simulink model "F16ASYM_Controlled_AoA"  (R2012b)
settings: Solver=ode3  SolverMode=SingleTasking  StartTime=0.0  StopTime=inf  FixedStep=T_sim  RelTol=1e-3
InitFcn:
  | load('NN_c_weights_Last_stable.mat')
values from neighbouring files (symbols this model uses):
  K_b_AoA = params(3)    [Cost_function.m]
  K_b_q = params(4)    [Cost_function.m]
  learning = 20    [Scheduling_desing.m]
  Model_used_flag = 1    [Scheduling_desing.m]
  reg_param = 0.5    [Scheduling_desing.m]
  T_sim = 0.02    [Scheduling_desing.m]
  tau_AoA = params(1)    [Cost_function.m]
  tau_q = params(2)    [Cost_function.m]
  Theta_1_roll_last = [0.00183613313267 0.00115998993235 0.0006676025148 0.00194921904952 0.00134963559861 0.00034352059664 0.000447169388141 0.00146749660935 0.00110199952389 7.77922383894e-05 0.00109492833348 0.00192687590535 ... (360 elements, 30x12)]    [NN_i_weights_LAST_STABLE.mat]
  Theta_2_roll_last = [0.000469743069697 0.000355923851088 0.00180035760697 0.00191855117771 0.00118851504447 0.0013331642065 0.0013164316578 0.000643981263341 0.00176817665434 0.000113802099363 0.000426534542462 0.00113815782354 ... (620 elements, 20x31)]    [NN_i_weights_LAST_STABLE.mat]
  Theta_3_roll_last = [9.62071520568e-05 -0.000389870886846 2.08260845013e-05 0.000140787743673 -0.000917525755397 -0.0014324207578 -0.00154701573815 -0.00131544476264 -0.00101205584381 5.06515794689e-05 -0.00111443483676 -0.00143957416141 ... (21 elements, 1x21)]    [NN_i_weights_LAST_STABLE.mat]
  V_long_lastA_w_z = [0.352826086601 -0.253633004548 -0.642535042878 0.237749930435 -0.618390629538 0.858074761295 0.268211230628 -0.448715080196 -0.0406384631192 0.401147605577 0.60598427709 0.0500551915851 ... (300 elements, 30x10)]    [NN_i_weights_LAST_STABLE.mat]
  V_long_lastAoA = [0.0774300162379 0.0911421319631 0.0352371192557 0.0542170286952 0.0651171200844 0.0177112012707 0.0982957728448 0.000259994642558 0.0194724569123 0.0466321328252 0.0556687953852 0.0252668067142 ... (300 elements, 30x10)]    [NN_i_weights_LAST_STABLE.mat]
  V_roll_last = [0.0540918675943 0.0557493347212 0.0839792276608 0.0460576391794 0.0671229058124 0.100220403067 0.0722493281881 0.0648875457457 0.00447599349201 0.0607299103823 0.0488037966361 0.0176785979393 ... (360 elements, 30x12)]    [NN_i_weights_LAST_STABLE.mat]
  V_yaw_last = [0.0965149149679 0.00833616709545 0.0365734360076 0.0523944217566 0.00790252078455 0.0700053845887 0.0345164868709 0.0111568465295 0.094060639546 0.0205483560006 0.000798047494256 0.0862769385758 ... (360 elements, 30x12)]    [NN_i_weights_LAST_STABLE.mat]
  velocity = M_eval_sche(I,J)*a    [Scheduling_desing.m]
  W_long_lastA_w_z = [-0.0522913429974 0.00385484301394 -0.00465489482472 -0.0139416219936 0.00295196421483 -0.013027768541 0.00585545058915 0.00278802233571 -0.00906272782329 -0.000396112031465 0.00405849743321 0.00509668457818 ... (31 elements, 1x31)]    [NN_i_weights_LAST_STABLE.mat]
  W_long_lastAoA = [-0.0192589013922 0.00873109909713 0.00432649597332 0.0420946902441 0.0293366820194 0.0351497798191 0.0234952374236 0.0360841187718 0.0112233388211 0.030147202199 0.0369533138617 0.00218839076415 ... (31 elements, 1x31)]    [NN_i_weights_LAST_STABLE.mat]
  W_roll_last = [-0.0006515532842 0.000535485585715 0.000550946920743 0.000806030945453 0.00045976209382 0.00065557954304 0.000945902185602 0.00070191398535 0.000635215543728 4.66501377412e-05 0.000597079583757 0.000485790566765 ... (31 elements, 1x31)]    [NN_i_weights_LAST_STABLE.mat]
  W_yaw_last = [-4.34263633305e-05 8.83823048922e-05 1.65575463724e-05 3.60293102233e-05 5.19752447623e-05 7.06399280852e-06 7.02425975821e-05 3.62680255076e-05 1.29996379937e-05 8.05072914397e-05 2.39941870661e-05 2.52427840574e-06 ... (31 elements, 1x31)]    [NN_i_weights_LAST_STABLE.mat]
undefined symbols (not defined in the file or in its folder): a1, alpha_map_eval, B, beta_map_eval, C_L_0, DiscIntNeverNeededParam, fi_flag_Simulink, G_eval, H_sq, H_sq_autotrim, k_B, m_B, M_sq, M_sq_autotrim, sigbuilder_block, Stall_curve, trim_control, trim_state, trim_throttle, V_Comp_A_w_z_last, V_Comp_last, V_roll_lastMOD, W_Comp_A_w_z_last, W_Comp_last, W_roll_lastMOD
libraries: Adaptive_FaultTolerantControl x43, dspsigops x29, F16_Actuator_Library x14, simulink x8, aerolibatmos2 x7, dsparch4 x6, simulink_extras x5, aerolibtransform2 x5, qcatlib x4, dspmtrx3 x3, dspvision x2, dspsnks4 x2
(part 7 of 11)

== system F16ASYM_Controlled_AoA/Control allocator/Control allocator: RECONFIG/Blockades logic: Limits injetor/Block AT SUPERIOR LIMIT ==
  Limit : Inport
  Blockades : Inport  Port=2
  Demux : Demux  Outputs=7
  Mux2 : Mux  Inputs=7
  Selector : Selector  InputPortWidth=7  IndexOptions=Index vector (dialog)  Indices=1  OutputSizes=1
  Selector1 : Selector  InputPortWidth=7  IndexOptions=Index vector (dialog)  Indices=2  OutputSizes=1
  Selector2 : Selector  InputPortWidth=7  IndexOptions=Index vector (dialog)  Indices=3  OutputSizes=1
  Selector3 : Selector  InputPortWidth=7  IndexOptions=Index vector (dialog)  Indices=4  OutputSizes=1
  Selector4 : Selector  InputPortWidth=7  IndexOptions=Index vector (dialog)  Indices=5  OutputSizes=1
  Selector5 : Selector  InputPortWidth=7  IndexOptions=Index vector (dialog)  Indices=6  OutputSizes=1
  Selector6 : Selector  InputPortWidth=7  IndexOptions=Index vector (dialog)  Indices=7  OutputSizes=1
  Switch{,1..6} (7 alike) : Switch  Threshold=0.5
  isNaN{,1..6} (7 alike) : RelationalOperator  Operator=isNaN  OutDataTypeStr=boolean
  Reconfig limits : Outport
  wires:
  Switch6/1 -> Mux2/7
  Switch5/1 -> Mux2/6  "LEF_L"
  Switch4/1 -> Mux2/5  "Rudder"
  Switch3/1 -> Mux2/4  "Aileron_R"
  Switch2/1 -> Mux2/3  "Aileron_L"
  Switch1/1 -> Mux2/2
  Switch/1 -> Mux2/1  "Elevator_L"
  Blockades/1 -> [Blockades]
  Mux2/1 -> Reconfig limits/1
  Limit/1 -> Demux/1
  Selector6/1 -> isNaN6/1, Switch6/3
  Demux/7 -> Switch6/1
  isNaN6/1 -> Switch6/2
  [Blockades] -> Selector6/1
  Selector5/1 -> isNaN5/1, Switch5/3
  Demux/6 -> Switch5/1
  isNaN5/1 -> Switch5/2
  [Blockades] -> Selector5/1
  Selector4/1 -> isNaN4/1, Switch4/3
  Demux/5 -> Switch4/1
  isNaN4/1 -> Switch4/2
  [Blockades] -> Selector4/1
  Selector3/1 -> isNaN3/1, Switch3/3
  Demux/4 -> Switch3/1
  isNaN3/1 -> Switch3/2
  [Blockades] -> Selector3/1
  Selector2/1 -> isNaN2/1, Switch2/3
  Demux/3 -> Switch2/1
  isNaN2/1 -> Switch2/2
  [Blockades] -> Selector2/1
  Selector1/1 -> isNaN1/1, Switch1/3
  Demux/2 -> Switch1/1
  isNaN1/1 -> Switch1/2
  [Blockades] -> Selector1/1
  Selector/1 -> isNaN/1, Switch/3
  Demux/1 -> Switch/1
  isNaN/1 -> Switch/2
  [Blockades] -> Selector/1

== system F16ASYM_Controlled_AoA/Control allocator/Control allocator: RECONFIG/Blockades logic: Limits injetor/Block NOW INFERIOR LIMIT ==
  Limit : Inport
  Blockade now : Inport  Port=2
  Last deflection (abs) : Inport  Port=3
  Demux : Demux  Outputs=7
  Mux2 : Mux  Inputs=7
  Selector1 : Selector  InputPortWidth=7  IndexOptions=Index vector (dialog)  Indices=1  OutputSizes=1
  Selector10 : Selector  InputPortWidth=7  IndexOptions=Index vector (dialog)  Indices=4  OutputSizes=1
  Selector11 : Selector  InputPortWidth=7  IndexOptions=Index vector (dialog)  Indices=5  OutputSizes=1
  Selector12 : Selector  InputPortWidth=7  IndexOptions=Index vector (dialog)  Indices=6  OutputSizes=1
  Selector13 : Selector  InputPortWidth=7  IndexOptions=Index vector (dialog)  Indices=7  OutputSizes=1
  Selector14 : Selector  InputPortWidth=7  IndexOptions=Index vector (dialog)  Indices=7  OutputSizes=1
  Selector2 : Selector  InputPortWidth=7  IndexOptions=Index vector (dialog)  Indices=2  OutputSizes=1
  Selector3 : Selector  InputPortWidth=7  IndexOptions=Index vector (dialog)  Indices=3  OutputSizes=1
  Selector4 : Selector  InputPortWidth=7  IndexOptions=Index vector (dialog)  Indices=4  OutputSizes=1
  Selector5 : Selector  InputPortWidth=7  IndexOptions=Index vector (dialog)  Indices=5  OutputSizes=1
  Selector6 : Selector  InputPortWidth=7  IndexOptions=Index vector (dialog)  Indices=6  OutputSizes=1
  Selector7 : Selector  InputPortWidth=7  IndexOptions=Index vector (dialog)  Indices=1  OutputSizes=1
  Selector8 : Selector  InputPortWidth=7  IndexOptions=Index vector (dialog)  Indices=2  OutputSizes=1
  Selector9 : Selector  InputPortWidth=7  IndexOptions=Index vector (dialog)  Indices=3  OutputSizes=1
  Switch{7..13} (7 alike) : Switch  Threshold=0.5
  Reconfig limits : Outport
  wires:
  Mux2/1 -> Reconfig limits/1
  Limit/1 -> Demux/1
  Selector13/1 -> Switch13/2
  [Blockade_now] -> Selector13/1
  Demux/7 -> Switch13/3
  Selector12/1 -> Switch12/2
  [Blockade_now] -> Selector12/1
  Demux/6 -> Switch12/3  "LEF_L"
  Selector11/1 -> Switch11/2
  [Blockade_now] -> Selector11/1
  Demux/5 -> Switch11/3  "Rudder"
  Selector10/1 -> Switch10/2
  [Blockade_now] -> Selector10/1
  Demux/4 -> Switch10/3  "Aileron_R"
  Selector9/1 -> Switch9/2
  [Blockade_now] -> Selector9/1
  Selector8/1 -> Switch8/2
  [Blockade_now] -> Selector8/1
  Demux/2 -> Switch8/3
  Selector7/1 -> Switch7/2
  [Blockade_now] -> Selector7/1
  Demux/1 -> Switch7/3  "Elevator_L"
  Blockade now/1 -> [Blockade_now]
  Last deflection (abs)/1 -> [Actual_defle]
  Demux/3 -> Switch9/3
  Switch7/1 -> Mux2/1
  Switch8/1 -> Mux2/2
  Switch9/1 -> Mux2/3
  Switch10/1 -> Mux2/4
  Switch11/1 -> Mux2/5
  Switch12/1 -> Mux2/6
  Switch13/1 -> Mux2/7
  [Actual_defle] -> Selector1/1
  Selector1/1 -> Switch7/1
  [Actual_defle] -> Selector2/1
  Selector2/1 -> Switch8/1
  Selector3/1 -> Switch9/1
  [Actual_defle] -> Selector3/1
  Selector4/1 -> Switch10/1
  [Actual_defle] -> Selector4/1
  Selector5/1 -> Switch11/1
  [Actual_defle] -> Selector5/1
  Selector6/1 -> Switch12/1
  [Actual_defle] -> Selector6/1
  Selector14/1 -> Switch13/1
  [Actual_defle] -> Selector14/1

== system F16ASYM_Controlled_AoA/Control allocator/Control allocator: RECONFIG/Blockades logic: Limits injetor/Block NOW SUPERIOR LIMIT ==
  Limit : Inport
  Blockade now : Inport  Port=2
  Last deflection (abs) : Inport  Port=3
  Demux : Demux  Outputs=7
  Mux2 : Mux  Inputs=7
  Selector1 : Selector  InputPortWidth=7  IndexOptions=Index vector (dialog)  Indices=1  OutputSizes=1
  Selector10 : Selector  InputPortWidth=7  IndexOptions=Index vector (dialog)  Indices=4  OutputSizes=1
  Selector11 : Selector  InputPortWidth=7  IndexOptions=Index vector (dialog)  Indices=5  OutputSizes=1
  Selector12 : Selector  InputPortWidth=7  IndexOptions=Index vector (dialog)  Indices=6  OutputSizes=1
  Selector13 : Selector  InputPortWidth=7  IndexOptions=Index vector (dialog)  Indices=7  OutputSizes=1
  Selector14 : Selector  InputPortWidth=7  IndexOptions=Index vector (dialog)  Indices=7  OutputSizes=1
  Selector2 : Selector  InputPortWidth=7  IndexOptions=Index vector (dialog)  Indices=2  OutputSizes=1
  Selector3 : Selector  InputPortWidth=7  IndexOptions=Index vector (dialog)  Indices=3  OutputSizes=1
  Selector4 : Selector  InputPortWidth=7  IndexOptions=Index vector (dialog)  Indices=4  OutputSizes=1
  Selector5 : Selector  InputPortWidth=7  IndexOptions=Index vector (dialog)  Indices=5  OutputSizes=1
  Selector6 : Selector  InputPortWidth=7  IndexOptions=Index vector (dialog)  Indices=6  OutputSizes=1
  Selector7 : Selector  InputPortWidth=7  IndexOptions=Index vector (dialog)  Indices=1  OutputSizes=1
  Selector8 : Selector  InputPortWidth=7  IndexOptions=Index vector (dialog)  Indices=2  OutputSizes=1
  Selector9 : Selector  InputPortWidth=7  IndexOptions=Index vector (dialog)  Indices=3  OutputSizes=1
  Switch{7..13} (7 alike) : Switch  Threshold=0.5
  Reconfig limits : Outport
  wires:
  [Actual_defle] -> Selector14/1
  Selector14/1 -> Switch13/1
  [Actual_defle] -> Selector6/1
  Selector6/1 -> Switch12/1
  [Actual_defle] -> Selector5/1
  Selector5/1 -> Switch11/1
  [Actual_defle] -> Selector4/1
  Selector4/1 -> Switch10/1
  [Actual_defle] -> Selector3/1
  Selector3/1 -> Switch9/1
  Selector2/1 -> Switch8/1
  [Actual_defle] -> Selector2/1
  Selector1/1 -> Switch7/1
  [Actual_defle] -> Selector1/1
  Switch13/1 -> Mux2/7
  Switch12/1 -> Mux2/6
  Switch11/1 -> Mux2/5
  Switch10/1 -> Mux2/4
  Switch9/1 -> Mux2/3
  Switch8/1 -> Mux2/2
  Switch7/1 -> Mux2/1
  Demux/3 -> Switch9/3
  Last deflection (abs)/1 -> [Actual_defle]
  Blockade now/1 -> [Blockade_now]
  Demux/1 -> Switch7/3  "Elevator_L"
  [Blockade_now] -> Selector7/1
  Selector7/1 -> Switch7/2
  Demux/2 -> Switch8/3
  [Blockade_now] -> Selector8/1
  Selector8/1 -> Switch8/2
  [Blockade_now] -> Selector9/1
  Selector9/1 -> Switch9/2
  Demux/4 -> Switch10/3  "Aileron_R"
  [Blockade_now] -> Selector10/1
  Selector10/1 -> Switch10/2
  Demux/5 -> Switch11/3  "Rudder"
  [Blockade_now] -> Selector11/1
  Selector11/1 -> Switch11/2
  Demux/6 -> Switch12/3  "LEF_L"
  [Blockade_now] -> Selector12/1
  Selector12/1 -> Switch12/2
  Demux/7 -> Switch13/3
  [Blockade_now] -> Selector13/1
  Selector13/1 -> Switch13/2
  Limit/1 -> Demux/1
  Mux2/1 -> Reconfig limits/1

== system F16ASYM_Controlled_AoA/Control allocator/Control allocator: RECONFIG/Leading Edge Flap:Symetric deflection/Creating    qbar // ps ==
  alt : Inport
  V : Inport  Port=2
  ISA Atmosphere Model : aerolibatmos2/ISA Atmosphere Model  custom=off  g=9.80665  gamma=1.4  R=287.0531  L=0.0065  h_trop=11000  h_strat=20000  rho0=1.225  P0=101325  T0=288.15
  Math Function1 : Math  Operator=square  SaturateOnIntegerOverflow=on
  Product : Product  Inputs=/*  SaturateOnIntegerOverflow=on  InputSameDT=on  OutDataTypeStr=Inherit: Same as first input
  Product5 : Product  Inputs=**  SaturateOnIntegerOverflow=on  InputSameDT=on  OutDataTypeStr=Inherit: Same as first input
  Terminator : Terminator
  Terminator1 : Terminator
  r2d4 : Gain  Gain=0.5  SaturateOnIntegerOverflow=on  OutDataTypeStr=Inherit: Same as input  ParamDataTypeStr=Inherit: Same as input
  qbar / ps : Outport
  wires:
  alt/1 -> ISA Atmosphere Model/1
  Math Function1/1 -> r2d4/1
  r2d4/1 -> Product5/2
  Product5/1 -> Product/2  "qbar"
  V/1 -> Math Function1/1
  Product/1 -> qbar / ps/1
  ISA Atmosphere Model/4 -> Product5/1
  ISA Atmosphere Model/3 -> Product/1
  ISA Atmosphere Model/1 -> Terminator/1
  ISA Atmosphere Model/2 -> Terminator1/1

== system F16ASYM_Controlled_AoA/Control allocator1/Control allocator: NO RECONF/Leading Edge Flap:Symetric deflection/Creating    qbar // ps ==
  alt : Inport
  V : Inport  Port=2
  ISA Atmosphere Model : aerolibatmos2/ISA Atmosphere Model  custom=off  g=9.80665  gamma=1.4  R=287.0531  L=0.0065  h_trop=11000  h_strat=20000  rho0=1.225  P0=101325  T0=288.15
  Math Function1 : Math  Operator=square  SaturateOnIntegerOverflow=on
  Product : Product  Inputs=/*  SaturateOnIntegerOverflow=on  InputSameDT=on  OutDataTypeStr=Inherit: Same as first input
  Product5 : Product  Inputs=**  SaturateOnIntegerOverflow=on  InputSameDT=on  OutDataTypeStr=Inherit: Same as first input
  Terminator : Terminator
  Terminator1 : Terminator
  r2d4 : Gain  Gain=0.5  SaturateOnIntegerOverflow=on  OutDataTypeStr=Inherit: Same as input  ParamDataTypeStr=Inherit: Same as input
  qbar / ps : Outport
  wires:
  ISA Atmosphere Model/2 -> Terminator1/1
  ISA Atmosphere Model/1 -> Terminator/1
  ISA Atmosphere Model/3 -> Product/1
  ISA Atmosphere Model/4 -> Product5/1
  Product/1 -> qbar / ps/1
  V/1 -> Math Function1/1
  Product5/1 -> Product/2  "qbar"
  r2d4/1 -> Product5/2
  Math Function1/1 -> r2d4/1
  alt/1 -> ISA Atmosphere Model/1

== system F16ASYM_Controlled_AoA/Control allocator1/Control allocator: RECONFIG/Blockades logic: Limits injetor/1st order model ==
  y_in : Inport
  Add : Sum  Inputs=|+-
  Integrator : Integrator  InitialCondition=y_i
  K_ref : Gain  Gain=K_ref
  y_out : Outport
  wires:
  Integrator/1 -> Add/2, y_out/1
  K_ref/1 -> Integrator/1
  Add/1 -> K_ref/1
  y_in/1 -> Add/1

== system F16ASYM_Controlled_AoA/Control allocator1/Control allocator: RECONFIG/Blockades logic: Limits injetor/1st order model1 ==
  y_in : Inport
  Add : Sum  Inputs=|+-
  Integrator : Integrator  InitialCondition=y_i
  K_ref : Gain  Gain=K_ref
  y_out : Outport
  wires:
  y_in/1 -> Add/1
  Add/1 -> K_ref/1
  K_ref/1 -> Integrator/1
  Integrator/1 -> y_out/1, Add/2

== system F16ASYM_Controlled_AoA/Control allocator1/Control allocator: RECONFIG/Blockades logic: Limits injetor/Block AT INFERIOR LIMIT ==
  Limit : Inport
  Blockades : Inport  Port=2
  Demux : Demux  Outputs=7
  Logical Operator : Logic  Operator=NOT  IconShape=distinctive  AllPortsSameDT=off  OutDataTypeStr=boolean
  Mux1 : Mux  Inputs=7
  Mux2 : Mux  Inputs=7
  Selector : Selector  InputPortWidth=7  IndexOptions=Index vector (dialog)  Indices=1  OutputSizes=1
  Selector1 : Selector  InputPortWidth=7  IndexOptions=Index vector (dialog)  Indices=2  OutputSizes=1
  Selector2 : Selector  InputPortWidth=7  IndexOptions=Index vector (dialog)  Indices=3  OutputSizes=1
  Selector3 : Selector  InputPortWidth=7  IndexOptions=Index vector (dialog)  Indices=4  OutputSizes=1
  Selector4 : Selector  InputPortWidth=7  IndexOptions=Index vector (dialog)  Indices=5  OutputSizes=1
  Selector5 : Selector  InputPortWidth=7  IndexOptions=Index vector (dialog)  Indices=6  OutputSizes=1
  Selector6 : Selector  InputPortWidth=7  IndexOptions=Index vector (dialog)  Indices=7  OutputSizes=1
  Switch{,1..6} (7 alike) : Switch  Threshold=0.5
  isNaN{,1..6} (7 alike) : RelationalOperator  Operator=isNaN  OutDataTypeStr=boolean
  Reconfig limits : Outport
  Surf blocked : Outport  Port=2
  wires:
  [Blockades] -> Selector/1
  isNaN/1 -> [left_elev], Switch/2
  Demux/1 -> Switch/1
  Selector/1 -> Switch/3, isNaN/1
  [Blockades] -> Selector1/1
  isNaN1/1 -> [right_elev], Switch1/2
  Demux/2 -> Switch1/1
  Selector1/1 -> Switch1/3, isNaN1/1
  [Blockades] -> Selector2/1
  isNaN2/1 -> Switch2/2, [left_ail]
  Demux/3 -> Switch2/1
  Selector2/1 -> Switch2/3, isNaN2/1
  [Blockades] -> Selector3/1
  isNaN3/1 -> [right_ail], Switch3/2
  Demux/4 -> Switch3/1
  Selector3/1 -> Switch3/3, isNaN3/1
  [Blockades] -> Selector4/1
  isNaN4/1 -> [rudder], Switch4/2
  Demux/5 -> Switch4/1
  Selector4/1 -> Switch4/3, isNaN4/1
  [Blockades] -> Selector5/1
  isNaN5/1 -> [left_LEF], Switch5/2
  Demux/6 -> Switch5/1
  Selector5/1 -> Switch5/3, isNaN5/1
  [Blockades] -> Selector6/1
  isNaN6/1 -> [rith_LEF], Switch6/2
  Demux/7 -> Switch6/1
  Selector6/1 -> Switch6/3, isNaN6/1
  Limit/1 -> Demux/1
  Mux2/1 -> Reconfig limits/1
  Blockades/1 -> [Blockades]
  Switch/1 -> Mux2/1  "Elevator_L"
  Switch1/1 -> Mux2/2
  Switch2/1 -> Mux2/3  "Aileron_L"
  Switch3/1 -> Mux2/4  "Aileron_R"
  Switch4/1 -> Mux2/5  "Rudder"
  Switch5/1 -> Mux2/6  "LEF_L"
  Switch6/1 -> Mux2/7
  [left_elev] -> Mux1/1
  Mux1/1 -> Logical Operator/1
  [right_elev] -> Mux1/2
  [left_ail] -> Mux1/3
  [right_ail] -> Mux1/4
  [rudder] -> Mux1/5
  [left_LEF] -> Mux1/6
  [rith_LEF] -> Mux1/7
  Logical Operator/1 -> Surf blocked/1

== system F16ASYM_Controlled_AoA/Control allocator1/Control allocator: RECONFIG/Blockades logic: Limits injetor/Block AT SUPERIOR LIMIT ==
  Limit : Inport
  Blockades : Inport  Port=2
  Demux : Demux  Outputs=7
  Mux2 : Mux  Inputs=7
  Selector : Selector  InputPortWidth=7  IndexOptions=Index vector (dialog)  Indices=1  OutputSizes=1
  Selector1 : Selector  InputPortWidth=7  IndexOptions=Index vector (dialog)  Indices=2  OutputSizes=1
  Selector2 : Selector  InputPortWidth=7  IndexOptions=Index vector (dialog)  Indices=3  OutputSizes=1
  Selector3 : Selector  InputPortWidth=7  IndexOptions=Index vector (dialog)  Indices=4  OutputSizes=1
  Selector4 : Selector  InputPortWidth=7  IndexOptions=Index vector (dialog)  Indices=5  OutputSizes=1
  Selector5 : Selector  InputPortWidth=7  IndexOptions=Index vector (dialog)  Indices=6  OutputSizes=1
  Selector6 : Selector  InputPortWidth=7  IndexOptions=Index vector (dialog)  Indices=7  OutputSizes=1
  Switch{,1..6} (7 alike) : Switch  Threshold=0.5
  isNaN{,1..6} (7 alike) : RelationalOperator  Operator=isNaN  OutDataTypeStr=boolean
  Reconfig limits : Outport
  wires:
  Switch6/1 -> Mux2/7
  Switch5/1 -> Mux2/6  "LEF_L"
  Switch4/1 -> Mux2/5  "Rudder"
  Switch3/1 -> Mux2/4  "Aileron_R"
  Switch2/1 -> Mux2/3  "Aileron_L"
  Switch1/1 -> Mux2/2
  Switch/1 -> Mux2/1  "Elevator_L"
  Blockades/1 -> [Blockades]
  Mux2/1 -> Reconfig limits/1
  Limit/1 -> Demux/1
  Selector6/1 -> isNaN6/1, Switch6/3
  Demux/7 -> Switch6/1
  isNaN6/1 -> Switch6/2
  [Blockades] -> Selector6/1
  Selector5/1 -> isNaN5/1, Switch5/3
  Demux/6 -> Switch5/1
  isNaN5/1 -> Switch5/2
  [Blockades] -> Selector5/1
  Selector4/1 -> isNaN4/1, Switch4/3
  Demux/5 -> Switch4/1
  isNaN4/1 -> Switch4/2
  [Blockades] -> Selector4/1
  Selector3/1 -> isNaN3/1, Switch3/3
  Demux/4 -> Switch3/1
  isNaN3/1 -> Switch3/2
  [Blockades] -> Selector3/1
  Selector2/1 -> isNaN2/1, Switch2/3
  Demux/3 -> Switch2/1
  isNaN2/1 -> Switch2/2
  [Blockades] -> Selector2/1
  Selector1/1 -> isNaN1/1, Switch1/3
  Demux/2 -> Switch1/1
  isNaN1/1 -> Switch1/2
  [Blockades] -> Selector1/1
  Selector/1 -> isNaN/1, Switch/3
  Demux/1 -> Switch/1
  isNaN/1 -> Switch/2
  [Blockades] -> Selector/1

== system F16ASYM_Controlled_AoA/Control allocator1/Control allocator: RECONFIG/Blockades logic: Limits injetor/Block NOW INFERIOR LIMIT ==
  Limit : Inport
  Blockade now : Inport  Port=2
  Last deflection (abs) : Inport  Port=3
  Demux : Demux  Outputs=7
  Mux2 : Mux  Inputs=7
  Sample and Hold{,1..7} (8 alike) : dspsigops/Sample and Hold  trig=Rising edge  initCond=trim_control(1)  latchinput=off
  Selector1 : Selector  InputPortWidth=7  IndexOptions=Index vector (dialog)  Indices=1  OutputSizes=1
  Selector10 : Selector  InputPortWidth=7  IndexOptions=Index vector (dialog)  Indices=4  OutputSizes=1
  Selector11 : Selector  InputPortWidth=7  IndexOptions=Index vector (dialog)  Indices=5  OutputSizes=1
  Selector12 : Selector  InputPortWidth=7  IndexOptions=Index vector (dialog)  Indices=6  OutputSizes=1
  Selector13 : Selector  InputPortWidth=7  IndexOptions=Index vector (dialog)  Indices=7  OutputSizes=1
  Selector14 : Selector  InputPortWidth=7  IndexOptions=Index vector (dialog)  Indices=7  OutputSizes=1
  Selector15 : Selector  InputPortWidth=7  IndexOptions=Index vector (dialog)  Indices=1  OutputSizes=1
  Selector2 : Selector  InputPortWidth=7  IndexOptions=Index vector (dialog)  Indices=2  OutputSizes=1
  Selector3 : Selector  InputPortWidth=7  IndexOptions=Index vector (dialog)  Indices=3  OutputSizes=1
  Selector4 : Selector  InputPortWidth=7  IndexOptions=Index vector (dialog)  Indices=4  OutputSizes=1
  Selector5 : Selector  InputPortWidth=7  IndexOptions=Index vector (dialog)  Indices=5  OutputSizes=1
  Selector6 : Selector  InputPortWidth=7  IndexOptions=Index vector (dialog)  Indices=6  OutputSizes=1
  Selector7 : Selector  InputPortWidth=7  IndexOptions=Index vector (dialog)  Indices=1  OutputSizes=1
  Selector8 : Selector  InputPortWidth=7  IndexOptions=Index vector (dialog)  Indices=2  OutputSizes=1
  Selector9 : Selector  InputPortWidth=7  IndexOptions=Index vector (dialog)  Indices=3  OutputSizes=1
  Switch{1,7..13} (8 alike) : Switch  Threshold=0.5
  Reconfig limits : Outport
  wires:
  Mux2/1 -> Reconfig limits/1
  Limit/1 -> Demux/1
  Selector13/1 -> Sample and Hold7/Trigger, Switch13/2
  [Blockade_now] -> Selector13/1
  Demux/7 -> Switch13/3
  Selector12/1 -> Switch12/2, Sample and Hold6/Trigger
  [Blockade_now] -> Selector12/1
  Demux/6 -> Switch12/3  "LEF_L"
  Selector11/1 -> Sample and Hold5/Trigger, Switch11/2
  [Blockade_now] -> Selector11/1
  Demux/5 -> Switch11/3  "Rudder"
  Selector10/1 -> Switch10/2, Sample and Hold4/Trigger
  [Blockade_now] -> Selector10/1
  Demux/4 -> Switch10/3  "Aileron_R"
  Selector9/1 -> Sample and Hold2/Trigger, Switch9/2
  [Blockade_now] -> Selector9/1
  Selector8/1 -> Sample and Hold3/Trigger, Switch8/2
  [Blockade_now] -> Selector8/1
  Demux/2 -> Switch8/3
  Selector7/1 -> Sample and Hold1/Trigger, Switch7/2
  [Blockade_now] -> Selector7/1
  Demux/1 -> Switch7/3  "Elevator_L"
  Blockade now/1 -> [Blockade_now]
  Last deflection (abs)/1 -> [Actual_defle]
  Demux/3 -> Switch9/3
  Switch7/1 -> Mux2/1
  Switch8/1 -> Mux2/2
  Switch9/1 -> Mux2/3
  Switch10/1 -> Mux2/4
  Switch11/1 -> Mux2/5
  Switch12/1 -> Mux2/6
  Switch13/1 -> Mux2/7
  [Actual_defle] -> Selector1/1
  Selector1/1 -> Sample and Hold1/1
  [Actual_defle] -> Selector2/1
  Selector2/1 -> Sample and Hold3/1
  Selector3/1 -> Sample and Hold2/1
  [Actual_defle] -> Selector3/1
  Selector4/1 -> Sample and Hold4/1
  [Actual_defle] -> Selector4/1
  Selector5/1 -> Sample and Hold5/1
  [Actual_defle] -> Selector5/1
  Sample and Hold6/1 -> Switch12/1
  [Actual_defle] -> Selector6/1
  Selector14/1 -> Sample and Hold7/1
  [Actual_defle] -> Selector14/1
  ? -> Switch1/3, Sample and Hold/1  "Elevator_L"
  [Blockade_now] -> Selector15/1
  Sample and Hold/1 -> Switch1/1
  Selector15/1 -> Switch1/2, Sample and Hold/Trigger
  Sample and Hold1/1 -> Switch7/1
  Sample and Hold2/1 -> Switch9/1
  Sample and Hold3/1 -> Switch8/1
  Sample and Hold4/1 -> Switch10/1
  Sample and Hold5/1 -> Switch11/1
  Selector6/1 -> Sample and Hold6/1
  Sample and Hold7/1 -> Switch13/1

== system F16ASYM_Controlled_AoA/Control allocator1/Control allocator: RECONFIG/Blockades logic: Limits injetor/Block NOW SUPERIOR LIMIT ==
  Limit : Inport
  Blockade now : Inport  Port=2
  Last deflection (abs) : Inport  Port=3
  Demux : Demux  Outputs=7
  Mux2 : Mux  Inputs=7
  Sample and Hold{,1..7} (8 alike) : dspsigops/Sample and Hold  trig=Rising edge  initCond=trim_control(1)  latchinput=off
  Selector1 : Selector  InputPortWidth=7  IndexOptions=Index vector (dialog)  Indices=1  OutputSizes=1
  Selector10 : Selector  InputPortWidth=7  IndexOptions=Index vector (dialog)  Indices=4  OutputSizes=1
  Selector11 : Selector  InputPortWidth=7  IndexOptions=Index vector (dialog)  Indices=5  OutputSizes=1
  Selector12 : Selector  InputPortWidth=7  IndexOptions=Index vector (dialog)  Indices=6  OutputSizes=1
  Selector13 : Selector  InputPortWidth=7  IndexOptions=Index vector (dialog)  Indices=7  OutputSizes=1
  Selector14 : Selector  InputPortWidth=7  IndexOptions=Index vector (dialog)  Indices=7  OutputSizes=1
  Selector15 : Selector  InputPortWidth=7  IndexOptions=Index vector (dialog)  Indices=1  OutputSizes=1
  Selector2 : Selector  InputPortWidth=7  IndexOptions=Index vector (dialog)  Indices=2  OutputSizes=1
  Selector3 : Selector  InputPortWidth=7  IndexOptions=Index vector (dialog)  Indices=3  OutputSizes=1
  Selector4 : Selector  InputPortWidth=7  IndexOptions=Index vector (dialog)  Indices=4  OutputSizes=1
  Selector5 : Selector  InputPortWidth=7  IndexOptions=Index vector (dialog)  Indices=5  OutputSizes=1
  Selector6 : Selector  InputPortWidth=7  IndexOptions=Index vector (dialog)  Indices=6  OutputSizes=1
  Selector7 : Selector  InputPortWidth=7  IndexOptions=Index vector (dialog)  Indices=1  OutputSizes=1
  Selector8 : Selector  InputPortWidth=7  IndexOptions=Index vector (dialog)  Indices=2  OutputSizes=1
  Selector9 : Selector  InputPortWidth=7  IndexOptions=Index vector (dialog)  Indices=3  OutputSizes=1
  Switch{1,7..13} (8 alike) : Switch  Threshold=0.5
  Reconfig limits : Outport
  wires:
  Sample and Hold7/1 -> Switch13/1
  Selector6/1 -> Sample and Hold6/1
  Sample and Hold5/1 -> Switch11/1
  Sample and Hold4/1 -> Switch10/1
  Sample and Hold3/1 -> Switch8/1
  Sample and Hold2/1 -> Switch9/1
  Sample and Hold1/1 -> Switch7/1
  Selector15/1 -> Sample and Hold/Trigger, Switch1/2
  Sample and Hold/1 -> Switch1/1
  [Blockade_now] -> Selector15/1
  ? -> Sample and Hold/1, Switch1/3  "Elevator_L"
  [Actual_defle] -> Selector14/1
  Selector14/1 -> Sample and Hold7/1
  [Actual_defle] -> Selector6/1
  Sample and Hold6/1 -> Switch12/1
  [Actual_defle] -> Selector5/1
  Selector5/1 -> Sample and Hold5/1
  [Actual_defle] -> Selector4/1
  Selector4/1 -> Sample and Hold4/1
  [Actual_defle] -> Selector3/1
  Selector3/1 -> Sample and Hold2/1
  Selector2/1 -> Sample and Hold3/1
  [Actual_defle] -> Selector2/1
  Selector1/1 -> Sample and Hold1/1
  [Actual_defle] -> Selector1/1
  Switch13/1 -> Mux2/7
  Switch12/1 -> Mux2/6
  Switch11/1 -> Mux2/5
  Switch10/1 -> Mux2/4
  Switch9/1 -> Mux2/3
  Switch8/1 -> Mux2/2
  Switch7/1 -> Mux2/1
  Demux/3 -> Switch9/3
  Last deflection (abs)/1 -> [Actual_defle]
  Blockade now/1 -> [Blockade_now]
  Demux/1 -> Switch7/3  "Elevator_L"
  [Blockade_now] -> Selector7/1
  Selector7/1 -> Switch7/2, Sample and Hold1/Trigger
  Demux/2 -> Switch8/3
  [Blockade_now] -> Selector8/1
  Selector8/1 -> Switch8/2, Sample and Hold3/Trigger
  [Blockade_now] -> Selector9/1
  Selector9/1 -> Switch9/2, Sample and Hold2/Trigger
  Demux/4 -> Switch10/3  "Aileron_R"
  [Blockade_now] -> Selector10/1
  Selector10/1 -> Sample and Hold4/Trigger, Switch10/2
  Demux/5 -> Switch11/3  "Rudder"
  [Blockade_now] -> Selector11/1
  Selector11/1 -> Switch11/2, Sample and Hold5/Trigger
  Demux/6 -> Switch12/3  "LEF_L"
  [Blockade_now] -> Selector12/1
  Selector12/1 -> Sample and Hold6/Trigger, Switch12/2
  Demux/7 -> Switch13/3
  [Blockade_now] -> Selector13/1
  Selector13/1 -> Switch13/2, Sample and Hold7/Trigger
  Limit/1 -> Demux/1
  Mux2/1 -> Reconfig limits/1

== system F16ASYM_Controlled_AoA/Control allocator1/Control allocator: RECONFIG/Leading Edge Flap:Symetric deflection/Creating    qbar // ps ==
  alt : Inport
  V : Inport  Port=2
  ISA Atmosphere Model : aerolibatmos2/ISA Atmosphere Model  custom=off  g=9.80665  gamma=1.4  R=287.0531  L=0.0065  h_trop=11000  h_strat=20000  rho0=1.225  P0=101325  T0=288.15
  Math Function1 : Math  Operator=square  SaturateOnIntegerOverflow=on
  Product : Product  Inputs=/*  SaturateOnIntegerOverflow=on  InputSameDT=on  OutDataTypeStr=Inherit: Same as first input
  Product5 : Product  Inputs=**  SaturateOnIntegerOverflow=on  InputSameDT=on  OutDataTypeStr=Inherit: Same as first input
  Terminator : Terminator
  Terminator1 : Terminator
  r2d4 : Gain  Gain=0.5  SaturateOnIntegerOverflow=on  OutDataTypeStr=Inherit: Same as input  ParamDataTypeStr=Inherit: Same as input
  qbar / ps : Outport
  wires:
  alt/1 -> ISA Atmosphere Model/1
  Math Function1/1 -> r2d4/1
  r2d4/1 -> Product5/2
  Product5/1 -> Product/2  "qbar"
  V/1 -> Math Function1/1
  Product/1 -> qbar / ps/1
  ISA Atmosphere Model/4 -> Product5/1
  ISA Atmosphere Model/3 -> Product/1
  ISA Atmosphere Model/1 -> Terminator/1
  ISA Atmosphere Model/2 -> Terminator1/1

== system F16ASYM_Controlled_AoA/F-16 Non-linear Plant/SYM and ASYM model: No reconfigurable/Leading Edge Flap:Symetric deflection/Creating    qbar // ps ==
  alt : Inport
  V : Inport  Port=2
  ISA Atmosphere Model : aerolibatmos2/ISA Atmosphere Model  custom=off  g=9.80665  gamma=1.4  R=287.0531  L=0.0065  h_trop=11000  h_strat=20000  rho0=1.225  P0=101325  T0=288.15
  Math Function1 : Math  Operator=square  SaturateOnIntegerOverflow=on
  Product : Product  Inputs=/*  SaturateOnIntegerOverflow=on  InputSameDT=on  OutDataTypeStr=Inherit: Same as first input
  Product5 : Product  Inputs=**  SaturateOnIntegerOverflow=on  InputSameDT=on  OutDataTypeStr=Inherit: Same as first input
  Terminator : Terminator
  Terminator1 : Terminator
  r2d4 : Gain  Gain=0.5  SaturateOnIntegerOverflow=on  OutDataTypeStr=Inherit: Same as input  ParamDataTypeStr=Inherit: Same as input
  qbar / ps : Outport
  wires:
  ISA Atmosphere Model/2 -> Terminator1/1
  ISA Atmosphere Model/1 -> Terminator/1
  ISA Atmosphere Model/3 -> Product/1
  ISA Atmosphere Model/4 -> Product5/1
  Product/1 -> qbar / ps/1
  V/1 -> Math Function1/1
  Product5/1 -> Product/2  "qbar"
  r2d4/1 -> Product5/2
  Math Function1/1 -> r2d4/1
  alt/1 -> ISA Atmosphere Model/1

== system F16ASYM_Controlled_AoA/F-16 Non-linear Plant/SYM and ASYM model: RECONFIGURABLE/Leading Edge Flap:Symetric deflection/Creating    qbar // ps ==
  alt : Inport
  V : Inport  Port=2
  ISA Atmosphere Model : aerolibatmos2/ISA Atmosphere Model  custom=off  g=9.80665  gamma=1.4  R=287.0531  L=0.0065  h_trop=11000  h_strat=20000  rho0=1.225  P0=101325  T0=288.15
  Math Function1 : Math  Operator=square  SaturateOnIntegerOverflow=on
  Product : Product  Inputs=/*  SaturateOnIntegerOverflow=on  InputSameDT=on  OutDataTypeStr=Inherit: Same as first input
  Product5 : Product  Inputs=**  SaturateOnIntegerOverflow=on  InputSameDT=on  OutDataTypeStr=Inherit: Same as first input
  Terminator : Terminator
  Terminator1 : Terminator
  r2d4 : Gain  Gain=0.5  SaturateOnIntegerOverflow=on  OutDataTypeStr=Inherit: Same as input  ParamDataTypeStr=Inherit: Same as input
  qbar / ps : Outport
  wires:
  alt/1 -> ISA Atmosphere Model/1
  Math Function1/1 -> r2d4/1
  r2d4/1 -> Product5/2
  Product5/1 -> Product/2  "qbar"
  V/1 -> Math Function1/1
  Product/1 -> qbar / ps/1
  ISA Atmosphere Model/4 -> Product5/1
  ISA Atmosphere Model/3 -> Product/1
  ISA Atmosphere Model/1 -> Terminator/1
  ISA Atmosphere Model/2 -> Terminator1/1

== system F16ASYM_Controlled_AoA/P controller + adaptive Crossed NN + AWU+Lim+scheduling   in AoA/Body Rates Controller/Ref Model and P Controller q/Reference Model ==
  y_ref : Inport
  Add : Sum  Inputs=|+-
  Integrator : Integrator  InitialCondition=trim_state(11)
  K_ref : Gain  Gain=1/tau_q
  y_c_dot : Outport
  y_c : Outport  Port=2
  wires:
  y_ref/1 -> Add/1
  Add/1 -> K_ref/1
  K_ref/1 -> Integrator/1, y_c_dot/1
  Integrator/1 -> y_c/1, Add/2

== system F16ASYM_Controlled_AoA/P controller + adaptive Crossed NN + AWU+Lim+scheduling   in AoA/Longitudinal controller in AoA/Ref Model and P Controller/Reference Model ==
  y_ref : Inport
  Add : Sum  Inputs=|+-
  Integrator : Integrator  InitialCondition=trim_state(8)
  K_ref : Gain  Gain=1/tau_AoA
  y_c_dot : Outport
  y_c : Outport  Port=2
  wires:
  y_ref/1 -> Add/1
  Add/1 -> K_ref/1
  K_ref/1 -> Integrator/1, y_c_dot/1
  Integrator/1 -> y_c/1, Add/2

== system F16ASYM_Controlled_AoA/Primary Controller/P  + Crossed NN + AWU+Lim + hand-over/P controller + adaptive Crossed NN + AWU+Lim    in ACC /Body Rates Controller ==
  p_ref : Inport
  q_ref : Inport  Port=2
  r_ref : Inport  Port=3
  All_meas : Inport  Port=4
  Bus Creator : BusCreator
  Bus Creator1 : BusCreator
  Bus Creator2 : BusCreator
  Bus Selector : BusSelector  OutputSignals=signal1.omega_b meas (rad/s)
  Display1 : Display
  Mux : Mux  Inputs=3
  Ref Model and P Controller p : Adaptive_FaultTolerantControl/Ref Model and P Controller  tau=0.1  y_i=trim_state(10)  K_f=1  K_b=7
  Ref Model and P Controller q : Adaptive_FaultTolerantControl/Ref Model and P Controller  tau=0.07  y_i=trim_state(11)  K_f=1  K_b=3
  Ref Model and P Controller r : Adaptive_FaultTolerantControl/Ref Model and P Controller  tau=0.2  y_i=trim_state(12)  K_f=1  K_b=4
  Selector : Selector  InputPortWidth=3  IndexOptions=Index vector (dialog)  Indices=1  OutputSizes=1
  Selector1 : Selector  InputPortWidth=3  IndexOptions=Index vector (dialog)  Indices=2  OutputSizes=1
  Selector2 : Selector  InputPortWidth=3  IndexOptions=Index vector (dialog)  Indices=3  OutputSizes=1
  Sum : Sum  Inputs=+-|
  Sum1 : Sum  Inputs=+-|
  Sum2 : Sum  Inputs=+-|
  q_chanel vars : Outport
  p_chanel vars : Outport  Port=2
  r_chanel vars : Outport  Port=3
  Angular acc des (rad/s^2) : Outport  Port=4
  wires:
  All_meas/1 -> Bus Selector/1
  Bus Selector/1 -> Selector/1, Selector1/1, Selector2/1  "<omega_b meas (rad/s)>"
  p_ref/1 -> Ref Model and P Controller p/1
  Selector/1 -> Ref Model and P Controller p/2
  Ref Model and P Controller p/1 -> Mux/1
  Mux/1 -> Angular acc des (rad/s^2)/1
  q_ref/1 -> Ref Model and P Controller q/1
  Selector1/1 -> Ref Model and P Controller q/2
  r_ref/1 -> Ref Model and P Controller r/1
  Ref Model and P Controller q/1 -> Mux/2
  Ref Model and P Controller r/1 -> Mux/3
  Ref Model and P Controller p/2 -> Bus Creator/1  "p_sf_dot"
  Ref Model and P Controller p/3 -> Sum/1, Bus Creator/2  "p_sf"
  Sum/1 -> Display1/1, Bus Creator/3  "p_err"
  Bus Creator/1 -> p_chanel vars/1
  Bus Creator1/1 -> q_chanel vars/1
  Bus Creator2/1 -> r_chanel vars/1
  Selector2/1 -> Ref Model and P Controller r/2
  Ref Model and P Controller p/4 -> Sum/2
  Ref Model and P Controller p/5 -> Bus Creator/4  "K_b_p"
  Ref Model and P Controller q/2 -> Bus Creator1/1  "q_sf_dot"
  Ref Model and P Controller q/3 -> Sum1/1, Bus Creator1/2  "q_sf"
  Sum1/1 -> Bus Creator1/3  "q_err"
  Ref Model and P Controller q/4 -> Sum1/2
  Ref Model and P Controller q/5 -> Bus Creator1/4  "K_b_q"
  Ref Model and P Controller r/2 -> Bus Creator2/1  "r_sf_dot"
  Ref Model and P Controller r/3 -> Sum2/1, Bus Creator2/2  "r_sf"
  Sum2/1 -> Bus Creator2/3  "r_err"
  Ref Model and P Controller r/4 -> Sum2/2
  Ref Model and P Controller r/5 -> Bus Creator2/4  "K_b_r"

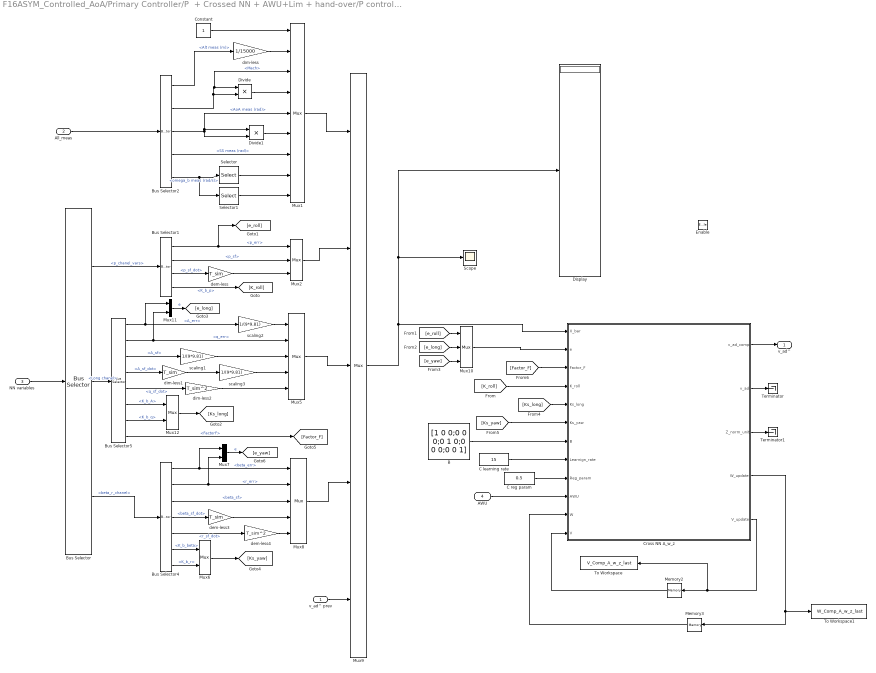
== system F16ASYM_Controlled_AoA/Primary Controller/P  + Crossed NN + AWU+Lim + hand-over/P controller + adaptive Crossed NN + AWU+Lim    in ACC /Complete crossed On-line (adaptive) multi-layer NN: A_w_z ==
  v_ad^ prev : Inport
  All_meas : Inport  Port=2
  NN variables : Inport  Port=3
  AWU : Inport  Port=4
  Enable : EnablePort  StatesWhenEnabling=reset
  B : Constant  Value=[1 0 0;0 0 0;0 1 0;0 0 0;0 0 1]
  Bus Selector : BusSelector  OutputSignals=p_chanel_vars,Long chanel,beta_r_chanel
  Bus Selector1 : BusSelector  OutputSignals=p_err,p_sf,p_sf_dot,K_b_p
  Bus Selector2 : BusSelector  OutputSignals=signal1.Alt meas (m),signal2.Mach,signal1.AoA meas (rad),signal1.SS meas (rad),signal1.omega_b meas (rad/s)
  Bus Selector4 : BusSelector  OutputSignals=beta_chanel vars.beta_err,r_chanel vars.r_err,beta_chanel vars.beta_sf,beta_chanel vars.beta_sf_dot,r_chanel vars.r_sf_dot,beta_chanel vars.K_b_beta,r_chanel vars.K_b_r
  Bus Selector5 : BusSelector  OutputSignals=A_chanel vars.A_err,q_chanel_vars.q_err,A_chanel vars.A_sf,A_chanel vars.A_sf_dot,q_chanel_vars.q_sf_dot,A_chanel vars.K_b_A,q_chanel_vars.K_b_q,A_chanel vars.FactorF
  C learning rate : Constant  Value=15  SampleTime=T_sim
  C reg param : Constant  Value=0.5  SampleTime=T_sim
  Constant : Constant
  Cross NN A_w_z : MATLAB Function  TreatAsAtomicUnit=on
  Display : Display
  Divide : Product  Inputs=**
  Divide1 : Product  Inputs=**
  Memory2 : Memory  X0=V_Comp_A_w_z_last
  Memory3 : Memory  X0=W_Comp_A_w_z_last
  Mux1 : Mux  Inputs=9
  Mux10 : Mux  Inputs=3
  Mux{6..7,11..12} (4 alike) : Mux  Inputs=2
  Mux2 : Mux  Inputs=3
  Mux5 : Mux  Inputs=5
  Mux8 : Mux  Inputs=5
  Mux9 : Mux  Inputs=[9 3 5 5 3]
  Scope : Scope
      settings: SaveName=ScopeData8
  Selector : Selector  InputPortWidth=3  IndexOptions=Index vector (dialog)  Indices=1  OutputSizes=1
  Selector1 : Selector  InputPortWidth=3  IndexOptions=Index vector (dialog)  Indices=3  OutputSizes=1
  Terminator : Terminator
  Terminator1 : Terminator
  To Workspace : ToWorkspace  VariableName=V_Comp_A_w_z_last  SampleTime=-1
      settings: MaxDataPoints=1
  To Workspace1 : ToWorkspace  VariableName=W_Comp_A_w_z_last  SampleTime=-1
      settings: MaxDataPoints=1
  dem-less : Gain  Gain=T_sim
  dem-less3 : Gain  Gain=T_sim
  dem-less4 : Gain  Gain=T_sim^2
  dim-less : Gain  Gain=1/15000
  dim-less1 : Gain  Gain=T_sim
  dim-less2 : Gain  Gain=T_sim^2
  scaling1 : Gain  Gain=1/(9*9.81)
  scaling2 : Gain  Gain=1/(9*9.81)
  scaling3 : Gain  Gain=1/(9*9.81)
  v_ad^ : Outport
  wires:
  [Factor_F] -> Cross NN A_w_z/3(Factor_F)
  Bus Selector5/8 -> [Factor_F]  "<FactorF>"
  scaling3/1 -> Mux5/4
  dim-less2/1 -> Mux5/5
  scaling1/1 -> Mux5/3
  Mux11/1 -> [e_long]  "e"
  Bus Selector/2 -> Bus Selector5/1  "<Long chanel>"
  Bus Selector5/1 -> Mux11/1, scaling2/1  "<A_err>"
  Bus Selector5/2 -> Mux11/2, Mux5/2  "<q_err>"
  Bus Selector5/3 -> scaling1/1  "<A_sf>"
  Bus Selector5/4 -> dim-less1/1  "<A_sf_dot>"
  Bus Selector5/5 -> dim-less2/1  "<q_sf_dot>"
  Bus Selector5/7 -> Mux12/2  "<K_b_q>"
  Bus Selector5/6 -> Mux12/1  "<K_b_A>"
  scaling2/1 -> Mux5/1
  dim-less1/1 -> scaling3/1
  Selector1/1 -> Mux1/9
  [Ks_yaw] -> Cross NN A_w_z/6(Ks_yaw)
  [Ks_long] -> Cross NN A_w_z/5(Ks_long)
  [K_roll] -> Cross NN A_w_z/4(K_roll)
  [e_yaw] -> Mux10/3
  [e_long] -> Mux10/2
  [e_roll] -> Mux10/1
  Mux10/1 -> Cross NN A_w_z/2(e)
  Cross NN A_w_z/4(W_update) -> To Workspace1/1, Memory3/1
  Cross NN A_w_z/5(V_update) -> Memory2/1, To Workspace/1
  Cross NN A_w_z/2(v_ad) -> Terminator/1
  B/1 -> Cross NN A_w_z/7(B)
  Memory3/1 -> Cross NN A_w_z/11(W)
  Memory2/1 -> Cross NN A_w_z/12(V)
  Cross NN A_w_z/1(v_ad_comp) -> v_ad^/1
  C learning rate/1 -> Cross NN A_w_z/8(Learnign_rate)
  C reg param/1 -> Cross NN A_w_z/9(Reg_param)
  Cross NN A_w_z/3(Z_norm_unit) -> Terminator1/1
  Mux9/1 -> Cross NN A_w_z/1(X_bar), Display/1, Scope/1
  v_ad^ prev/1 -> Mux9/5
  Mux8/1 -> Mux9/4
  Mux5/1 -> Mux9/3
  Mux2/1 -> Mux9/2
  Mux1/1 -> Mux9/1
  dem-less4/1 -> Mux8/5
  Mux7/1 -> [e_yaw]  "e"
  Bus Selector4/2 -> Mux7/2, Mux8/2  "<r_err>"
  Bus Selector4/1 -> Mux7/1, Mux8/1  "<beta_err>"
  Mux6/1 -> [Ks_yaw]
  Bus Selector4/6 -> Mux6/1  "<K_b_beta>"
  Bus Selector4/7 -> Mux6/2  "<K_b_r>"
  Bus Selector4/5 -> dem-less4/1  "<r_sf_dot>"
  Bus Selector4/4 -> dem-less3/1  "<beta_sf_dot>"
  Bus Selector4/3 -> Mux8/3  "<beta_sf>"
  dem-less3/1 -> Mux8/4
  Mux12/1 -> [Ks_long]
  dem-less/1 -> Mux2/3
  Bus Selector1/1 -> Mux2/1, [e_roll]  "<p_err>"
  Bus Selector1/2 -> Mux2/2  "<p_sf>"
  Bus Selector1/4 -> [K_roll]  "<K_b_p>"
  Bus Selector2/3 -> Divide1/2, Mux1/5, Divide1/1  "<AoA meas (rad)>"
  Bus Selector2/2 -> Divide/1, Mux1/3, Divide/2  "<Mach>"
  Bus Selector2/4 -> Mux1/7  "<SS meas (rad)>"
  Selector/1 -> Mux1/8
  Bus Selector1/3 -> dem-less/1  "<p_sf_dot>"
  Constant/1 -> Mux1/1
  All_meas/1 -> Bus Selector2/1
  Bus Selector2/1 -> dim-less/1  "<Alt meas (m)>"
  Divide/1 -> Mux1/4
  Divide1/1 -> Mux1/6
  dim-less/1 -> Mux1/2
  Bus Selector2/5 -> Selector/1, Selector1/1  "<omega_b meas (rad/s)>"
  NN variables/1 -> Bus Selector/1
  Bus Selector/1 -> Bus Selector1/1  "<p_chanel_vars>"
  Bus Selector/3 -> Bus Selector4/1  "<beta_r_chanel>"
  AWU/1 -> Cross NN A_w_z/10(AWU)

== system F16ASYM_Controlled_AoA/Primary Controller/P  + Crossed NN + AWU+Lim + hand-over/P controller + adaptive Crossed NN + AWU+Lim    in ACC /Lat_dir Dyn Inversion: beta_dot->r_c ==
  beta_dot_c : Inport
  All_meas : Inport  Port=2
  A_w_y : Selector  InputPortWidth=3  IndexOptions=Index vector (dialog)  Indices=2  OutputSizes=1
  Bus Selector : BusSelector  OutputSignals=signal1.AoA meas (rad),signal1.omega_b meas (rad/s),signal1.V_TAS (m/s),signal2.A_w_CG
  Divide1 : Product  Inputs=**
  Divide3 : Product  Inputs=**
  Divide4 : Product  Inputs=/*
  Divide5 : Product  Inputs=*/
  Selector : Selector  InputPortWidth=3  IndexOptions=Index vector (dialog)  Indices=1  OutputSizes=1
  Trigonometric Function : Trigonometry  Operator=cos
  Trigonometric Function3 : Trigonometry  Operator=tan
  "q_c " : Sum  Inputs=-++
  r_c : Outport
  wires:
  "q_c "/1 -> r_c/1
  Bus Selector/1 -> Trigonometric Function/1, Trigonometric Function3/1  "<AoA meas (rad)>"
  Bus Selector/2 -> Selector/1  "<omega_b meas (rad/s)>"
  Divide1/1 -> "q_c "/2
  Divide3/1 -> Divide4/1
  A_w_y/1 -> Divide4/2
  All_meas/1 -> Bus Selector/1
  Bus Selector/4 -> A_w_y/1  "<A_w_CG>"
  Divide4/1 -> "q_c "/3
  Bus Selector/3 -> Divide3/2  "<V_TAS (m/s)>"
  Trigonometric Function/1 -> Divide3/1, Divide5/2
  Divide5/1 -> "q_c "/1
  beta_dot_c/1 -> Divide5/1
  Trigonometric Function3/1 -> Divide1/1
  Selector/1 -> Divide1/2

== system F16ASYM_Controlled_AoA/Primary Controller/P  + Crossed NN + AWU+Lim + hand-over/P controller + adaptive Crossed NN + AWU+Lim    in ACC /Long Dyn Inversion: alpha_dot ->q ==
  alpha_dot_c : Inport
  All_meas : Inport  Port=2
  Completed : Subsystem
  Manual Switch : ManualSwitch
  Simplified : Subsystem
  q_c : Outport
  wires:
  alpha_dot_c/1 -> Simplified/1(alpha_dot_c), Completed/1(alpha_dot_c)
  All_meas/1 -> Simplified/2(All_meas), Completed/2(All_meas)
  Completed/1(q_c) -> Manual Switch/1
  Simplified/1(q_c) -> Manual Switch/2
  Manual Switch/1 -> q_c/1

== system F16ASYM_Controlled_AoA/Primary Controller/P  + Crossed NN + AWU+Lim + hand-over/P controller + adaptive Crossed NN + AWU+Lim    in ACC /Longitudinal controller in A_w_z ==
  A_w_z des : Inport
  AoA des (rad) : Inport  Port=2
  Anti-windup A_w_z : Inport  Port=3
  Anti-windup AoA : Inport  Port=4
  All meas : Inport  Port=5
  Accel rate --> AoA rate! : Subsystem
  Bus Creator : BusCreator  Inputs=5
  Bus Selector : BusSelector  OutputSignals=signal2.A_w_CG
  Divide : Product  Inputs=**
  Gain : Gain  Gain=-1
  Ref Model and P Controller : Adaptive_FaultTolerantControl/Ref Model and P Controller  tau=0.3  y_i=0  K_f=1  K_b=2.5
  Selector : Selector  InputPortWidth=3  IndexOptions=Index vector (dialog)  Indices=3  OutputSizes=1
  Stall protection : Subsystem  Commented=on
  Sum : Sum  Inputs=+-|
  Terminator : Terminator
  Terminator1 : Terminator
  Terminator2 : Terminator
  A_chanel vars : Outport
  alpha_dot_c : Outport  Port=2
  wires:
  Anti-windup AoA/1 -> Terminator1/1
  AoA des (rad)/1 -> Terminator/1
  Selector/1 -> Gain/1
  Gain/1 -> Ref Model and P Controller/2
  Bus Selector/1 -> Selector/1  "<A_w_CG>"
  Anti-windup A_w_z/1 -> Terminator2/1
  A_w_z des/1 -> Ref Model and P Controller/1
  Ref Model and P Controller/1 -> Divide/1
  Ref Model and P Controller/2 -> Bus Creator/1  "A_sf_dot"
  Ref Model and P Controller/3 -> Bus Creator/2, Sum/1  "A_sf"
  Sum/1 -> Bus Creator/3  "A_err"
  Ref Model and P Controller/4 -> Sum/2
  Ref Model and P Controller/5 -> Bus Creator/4  "K_b_A"
  Bus Creator/1 -> A_chanel vars/1
  Divide/1 -> alpha_dot_c/1
  Accel rate --> AoA rate!/1(A_w  to AoA rates factor) -> Bus Creator/5, Divide/2  "FactorF"
  All meas/1 -> Bus Selector/1, Stall protection/2(All meas), Accel rate --> AoA rate!/1(All_meas)

== system F16ASYM_Controlled_AoA/Primary Controller/P  + Crossed NN + AWU+Lim + hand-over/P controller + adaptive Crossed NN + AWU+Lim    in ACC /Physical limitation ==
  note: Converto to Angular accelerations
  v comm : Inport
  all meas : Inport  Port=2
  Ang Accel : MATLAB Function
  Bus Selector : BusSelector  OutputSignals=signal1.Alt meas (m),signal1.V_TAS (m/s),signal1.AoA meas (rad),signal1.SS meas (rad),signal1.omega_b meas (rad/s),signal1.Throttle_meas
  Bus Selector1 : BusSelector  OutputSignals=signal2.q (Pa),signal1.omega_b meas (rad/s)
  Demux : Demux  Outputs=3
  Display : Display
  Display1 : Display
  Display2 : Display
  Divide : Product  Inputs=**
  Divide1 : Product  Inputs=**
  Gain : Gain  Gain=-1
  Gain1 : Gain
  Mom coefficients that was reached : MATLABFcn  MATLABFcn=Moms_Coeff_estimator  OutputDimensions=3  OutputSignalType=real
  Moments : Subsystem
  Mux : Mux  Inputs=3
  Mux1 : Mux  Inputs=7
  Saturation Dynamic : simulink/Discontinuities/Saturation Dynamic  OutMin=[]  OutMax=[]  OutDataTypeStr=Inherit: Same as second input  OutDataType=fixdt(1, 16)  OutScaling=2^-10  DoSatur=off
  Sign : Signum
  Sign1 : Signum
  max deflections estimator : MATLAB Function  TreatAsAtomicUnit=on
  v limted : Outport
  wires:
  max deflections estimator/1(max_defl) -> Mux1/7
  Mux1/1 -> Mom coefficients that was reached/1
  Bus Selector/5 -> Mux1/5  "<omega_b meas (rad/s)>"
  Bus Selector/1 -> Mux1/1  "<Alt meas (m)>"
  Bus Selector/2 -> Mux1/2  "<V_TAS (m/s)>"
  Bus Selector/3 -> Mux1/3  "<AoA meas (rad)>"
  Bus Selector/4 -> Mux1/4  "<SS meas (rad)>"
  Bus Selector/6 -> Mux1/6  "<Throttle_meas>"
  Ang Accel/2(q_dot) -> Mux/2
  Ang Accel/3(r_dot) -> Mux/3
  Ang Accel/1(p_dot) -> Mux/1
  Bus Selector1/2 -> Ang Accel/4(omega_b)  "<omega_b meas (rad/s)>"
  Moments/3(N) -> Ang Accel/3(N)
  Moments/2(M) -> Ang Accel/2(M)
  Moments/1(L) -> Ang Accel/1(L)
  Bus Selector1/1 -> Moments/4(q)  "<q (Pa)>"
  Demux/3 -> Moments/3(C_N)
  Demux/2 -> Moments/2(C_M)
  Demux/1 -> Moments/1(C_L)
  Mom coefficients that was reached/1 -> Demux/1
  all meas/1 -> Bus Selector/1, Bus Selector1/1
  Mux/1 -> Gain1/1
  v comm/1 -> Saturation Dynamic/2, Display1/1, max deflections estimator/1(v_comm)
  Saturation Dynamic/1 -> Display/1, v limted/1
  Sign/1 -> Divide/1
  Gain1/1 -> Divide/2, Divide1/1, Sign1/1, Display2/1, Sign/1
  Sign1/1 -> Gain/1
  Divide/1 -> Saturation Dynamic/1
  Gain/1 -> Divide1/2
  Divide1/1 -> Saturation Dynamic/3

== system F16ASYM_Controlled_AoA/Primary Controller/P  + Crossed NN + AWU+Lim + hand-over/P controller + adaptive Crossed NN + AWU+Lim    in ACC /Sigmoid  ==
  In : Inport
  Display : Display
  Fcn1 : Fcn  Commented=on  Expr=2.0 ./ (1.0 + exp(-u(4)*u(1:3)))-1
  MATLAB Function : MATLAB Function  TreatAsAtomicUnit=on
  a : Constant  Value=a
  Out : Outport
  wires:
  MATLAB Function/1(y) -> Display/1, Out/1
  In/1 -> MATLAB Function/1(u)
  a/1 -> MATLAB Function/2(a)

== matlab function F16ASYM_Controlled_AoA/Primary Controller/P controller + adaptive Crossed NN + AWU+Lim /Longitudinal Controller: AoA or A_w_z/Longitudinal controller in A_w_z/Stall protection/MATLAB Function ==
  data: alpha_dot input; alpha_dot_out output; alpha input
function alpha_dot_out = AoA_limit(alpha_dot,alpha)
a=180/pi;
AoA_sup = deg2rad(18);
AoA_inf = -deg2rad(18);


if (alpha>0 & alpha_dot<0)  || (alpha<0 & alpha_dot>0) 
    alpha_dot_out = alpha_dot;
else
    alpha_dot_out  = ( 2./(1+exp(-a*(alpha-AoA_inf ))) -1 -2./(1+exp(-a*(alpha-AoA_sup ))) )*alpha_dot;
end

== matlab function F16ASYM_Controlled_AoA/Primary Controller/P  + Crossed NN + AWU+Lim + hand-over/P controller + adaptive Crossed NN + AWU+Lim   in AoA/Sigmoid /MATLAB Function ==
  data: u input; y output; a input
function y = sigmoid_a(u,a)

y = 2.0 ./ (1.0 + exp(-a*u(1:3)))-1;
